simulink library "SimplusGT_2020a"  (R2021a)
settings: Solver=ode45  StartTime=0.0  StopTime=10.0  RelTol=1e-3
undefined symbols (not defined in the file): ang_r, Cf, DiscIntNeverNeededParam, initial, Lc, Lf, m, OtherInputs, P_dc, Sbase, t0, Tm_pu, Ts, V, Vbase, w_droop, w_i, w_pll, w_tau, w_v, Wbase, wc, wfil, x0, Ybase, Zbase
libraries: spsVoltageMeasurementLib x83, spsCurrentMeasurementLib x71, spsControlledCurrentSourceLib x33, spsThreePhaseSeriesRLCBranchLib x21, spsControlledVoltageSourceLib x19, spsSeriesRLCBranchLib x15, spsThreePhaseParallelRLCBranchLib x3, spsThreePhaseBreakerLib x2, $bdroot x1, SimplexPS_2015a x1
(part 3 of 6)

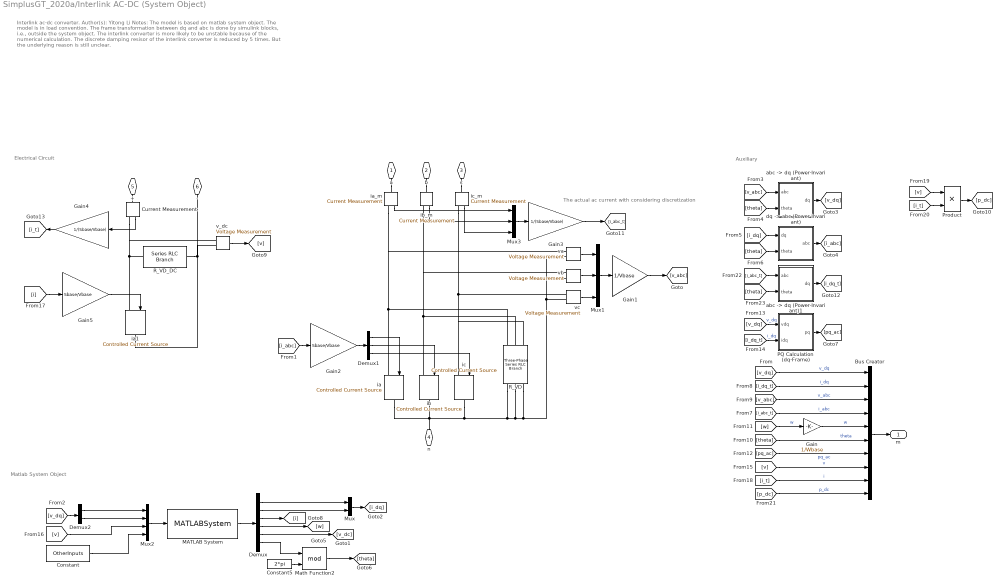
== system SimplusGT_2020a/Interlink AC-DC (System Object) ==
  note: Matlab System Object
  note: Auxiliary
  note: Electrical Circuit
  note: Interlink ac-dc converter.
      |
      | Author(s): Yitong Li
      |
      | Notes:
      |
      | The model is based on matlab system object.
      |
      | The model is in load convention.
      |
      | The frame transformation between dq and abc is done by simulink blocks, i.e., outside the system object.
      |
      | The interlink converter is more likely to be unstable because of the numerical calculation. The discrete damping resisor of the interlink converter is reduced by 5 times. But the underlying reason is still unclear.
  note: The actual ac current with considering discretization
  Bus Creator : BusCreator  Inputs=10
  Constant : Constant  Value=OtherInputs
  Constant5 : Constant  Value=2*pi
  Current Measurement : spsCurrentMeasurementLib/Current Measurement  PhasorSimulation=off  OutputType=Complex  PSBequivalent=0
  Demux : Demux  Outputs=6
  Demux1 : Demux  Outputs=3
  Demux2 : Demux  Outputs=2
  Gain : Gain  Gain=1/Wbase
  Gain1 : Gain  Gain=1/Vbase
  Gain2 : Gain  Gain=Sbase/Vbase
  Gain3 : Gain  Gain=1/(Sbase/Vbase)
  Gain4 : Gain  Gain=1/(Sbase/Vbase)
  Gain5 : Gain  Gain=Sbase/Vbase
  MATLAB System : MATLABSystem  System=SimplusGT.Class.InterlinkAcDc  Ts=Ts  Para=ApparatusPara  ApparatusType=ApparatusType  PowerFlow=PowerFlow  x0=x0  DiscreMethod=DiscreMethod  LinearizationTimes=LinearizationTimes  DirectFeedthrough=DirectFeedthrough  VirtualResistor=DiscreDampingFlag  EquiInitial=true  ElecPortIOs=[ 1, 2, 3 ]  SimulateUsing=Code generation
      mask Type: SimplusGT.Class.InterlinkAcDc
      mask Display:
      | disp('InterlinkAcDc');
      | port_label('input',1,'u');
      | port_label('output',1,'y');
  Math Function2 : Math  Operator=mod  SignedPower=on  SaturateOnIntegerOverflow=on
  Mux : Mux  Inputs=2
  Mux1 : Mux  Inputs=3
  Mux2 : Mux
  Mux3 : Mux  Inputs=3
  PQ Calculation (dq-Frame) : Subsystem  AncestorBlock=|
      | SimplusGT/PQ Calculation
      | (dq-Frame)
  Product : Product
  R_VD : spsThreePhaseSeriesRLCBranchLib/Three-Phase Series RLC Branch  LConnTagsString=A|B|C  RConnTagsString=A|B|C  BranchType=R  Resistance=DiscreDampingValue*Vbase^2/Sbase/5  Inductance=1e-3  Capacitance=1e-6  Measurements=None
  R_VD_DC : spsSeriesRLCBranchLib/Series RLC Branch  LConnTagsString=__new0  RConnTagsString=__new0  BranchType=R  Resistance=DiscreDampingValue*Vbase^2/Sbase/5  Inductance=1e-3  SetiL0=off  InitialCurrent=0  Capacitance=1e-6  Setx0=off  InitialVoltage=0  Measurements=None
  "abc -> dq (Power-Invariant)" : Subsystem  AncestorBlock=|
      | SimplusGT/abc -> dq
      | (Power-Invariant)
  "abc -> dq (Power-Invariant)1" : Subsystem  AncestorBlock=|
      | SimplusGT/abc -> dq
      | (Power-Invariant)
  "dq -> abc (Power-Invariant)" : Subsystem  AncestorBlock=|
      | SimplusGT/dq -> abc
      | (Power-Invariant)
  ia : spsControlledCurrentSourceLib/Controlled Current Source  Initialize=on  Source_Type=AC  Amplitude=0  Phase=0  Frequency=0  Measurements=None
  ia1 : spsControlledCurrentSourceLib/Controlled Current Source  Initialize=on  Source_Type=AC  Amplitude=0  Phase=0  Frequency=0  Measurements=None
  ia_m : spsCurrentMeasurementLib/Current Measurement  PhasorSimulation=off  OutputType=Complex  PSBequivalent=0
  ib : spsControlledCurrentSourceLib/Controlled Current Source  Initialize=on  Source_Type=AC  Amplitude=0  Phase=0  Frequency=0  Measurements=None
  ib_m : spsCurrentMeasurementLib/Current Measurement  PhasorSimulation=off  OutputType=Complex  PSBequivalent=0
  ic : spsControlledCurrentSourceLib/Controlled Current Source  Initialize=on  Source_Type=AC  Amplitude=0  Phase=0  Frequency=0  Measurements=None
  ic_m : spsCurrentMeasurementLib/Current Measurement  PhasorSimulation=off  OutputType=Complex  PSBequivalent=0
  v_dc : spsVoltageMeasurementLib/Voltage Measurement  PhasorSimulation=off  OutputType=Complex  PSBequivalent=0
  va : spsVoltageMeasurementLib/Voltage Measurement  PhasorSimulation=off  OutputType=Complex  PSBequivalent=0
  vb : spsVoltageMeasurementLib/Voltage Measurement  PhasorSimulation=off  OutputType=Complex  PSBequivalent=0
  vc : spsVoltageMeasurementLib/Voltage Measurement  PhasorSimulation=off  OutputType=Complex  PSBequivalent=0
  a : PMIOPort  Side=Left
  b : PMIOPort  Port=2  Side=Left
  c : PMIOPort  Port=3  Side=Left
  n : PMIOPort  Port=4  Side=Left
  + : PMIOPort  Port=5  Side=Left
  - : PMIOPort  Port=6  Side=Left
  m : Outport
  wires:
  Demux/2 -> Mux/2
  Demux/1 -> Mux/1
  Mux/1 -> [i_dq]
  Demux1/1 -> ia/1
  Demux1/2 -> ib/1
  va/1 -> Mux1/1
  vb/1 -> Mux1/2
  Mux1/1 -> Gain1/1
  [v_dq] -> Demux2/1
  Demux2/1 -> Mux2/1
  Demux2/2 -> Mux2/2
  [v_dq] -> Bus Creator/1  "v_dq"
  [i_dq_t] -> Bus Creator/2  "i_dq"
  [v_abc] -> Bus Creator/3  "v_abc"
  [i_abc_t] -> Bus Creator/4  "i_abc"
  [theta] -> Bus Creator/6  "theta"
  [v_abc] -> "abc -> dq (Power-Invariant)"/1(abc)
  [theta] -> "abc -> dq (Power-Invariant)"/2(theta)
  "abc -> dq (Power-Invariant)"/1(dq) -> [v_dq]
  [i_dq] -> "dq -> abc (Power-Invariant)"/1(dq)
  [theta] -> "dq -> abc (Power-Invariant)"/2(theta)
  "dq -> abc (Power-Invariant)"/1(abc) -> [i_abc]
  Mux2/1 -> MATLAB System/1
  MATLAB System/1 -> Demux/1
  vc/1 -> Mux1/3
  Demux1/3 -> ic/1
  Constant5/1 -> Math Function2/2
  Math Function2/1 -> [theta]
  Bus Creator/1 -> m/1
  Constant/1 -> Mux2/4
  [w] -> Gain/1  "w"
  Gain/1 -> Bus Creator/5  "w"
  [i_abc] -> Gain2/1
  [pq_ac] -> Bus Creator/7  "pq_ac"
  [v_dq] -> PQ Calculation (dq-Frame)/1(vdq)  "v_dq"
  [i_dq_t] -> PQ Calculation (dq-Frame)/2(idq)  "i_dq"
  PQ Calculation (dq-Frame)/1(pq) -> [pq_ac]
  Gain2/1 -> Demux1/1
  Gain1/1 -> [v_abc]
  [v] -> Bus Creator/8  "v"
  Demux/4 -> [w]
  Demux/5 -> [v_dc]
  Demux/6 -> Math Function2/1
  [v] -> Mux2/3
  Demux/3 -> [i]
  v_dc/1 -> [v]
  [i_t] -> Bus Creator/9  "i"
  [v] -> Product/1
  [i_t] -> Product/2
  Product/1 -> [p_dc]
  [p_dc] -> Bus Creator/10  "p_dc"
  ic_m/1 -> Mux3/3
  ib_m/1 -> Mux3/2
  Gain3/1 -> [i_abc_t]
  Mux3/1 -> Gain3/1
  ia_m/1 -> Mux3/1
  [theta] -> "abc -> dq (Power-Invariant)1"/2(theta)
  [i_abc_t] -> "abc -> dq (Power-Invariant)1"/1(abc)
  "abc -> dq (Power-Invariant)1"/1(dq) -> [i_dq_t]
  Gain4/1 -> [i_t]
  Current Measurement/1 -> Gain4/1
  [i] -> Gain5/1
  Gain5/1 -> ia1/1
  connections:
  vb/LConn2 -- va/LConn2 -- vc/LConn2 -- R_VD/RConn3 -- R_VD/RConn2 -- R_VD/RConn1 -- ic/RConn1 -- ia/RConn1 -- ib/RConn1 -- n/RConn1
  R_VD/LConn1 -- ia_m/RConn1 -- va/LConn1 -- ia/LConn1
  R_VD/LConn2 -- ib_m/RConn1 -- vb/LConn1 -- ib/LConn1
  R_VD/LConn3 -- ic/LConn1 -- ic_m/RConn1 -- vc/LConn1
  ia1/LConn1 -- Current Measurement/RConn1 -- v_dc/LConn1 -- R_VD_DC/LConn1
  ia1/RConn1 -- R_VD_DC/RConn1 -- -/RConn1 -- v_dc/LConn2
  c/RConn1 -- ic_m/LConn1
  b/RConn1 -- ib_m/LConn1
  a/RConn1 -- ia_m/LConn1
  Current Measurement/LConn1 -- +/RConn1

== system SimplusGT_2020a/L Filter (3ph) ==
  note: Model for a L filter.
      |
      | Author(s): Yitong Li
      |
      | Notes:
      |
      | vi is the converter side voltage, and vg is the grid side voltage.
  Bus Creator : BusCreator  Inputs=3
  "LL -> LN" : Subsystem
  "LL -> LN1" : Subsystem
  Mux : Mux  Inputs=3
  Mux1 : Mux  Inputs=3
  Mux2 : Mux  Inputs=3
  Three-Phase Series RLC Branch : spsThreePhaseSeriesRLCBranchLib/Three-Phase Series RLC Branch  LConnTagsString=A|B|C  RConnTagsString=A|B|C  BranchType=RL  Resistance=Rf  Inductance=Lf  Capacitance=1e-6  Measurements=None
  Vab : spsVoltageMeasurementLib/Voltage Measurement  PhasorSimulation=off  OutputType=Complex  PSBequivalent=0
  Vab1 : spsVoltageMeasurementLib/Voltage Measurement  PhasorSimulation=off  OutputType=Complex  PSBequivalent=0
  Vbc : spsVoltageMeasurementLib/Voltage Measurement  PhasorSimulation=off  OutputType=Complex  PSBequivalent=0
  Vbc1 : spsVoltageMeasurementLib/Voltage Measurement  PhasorSimulation=off  OutputType=Complex  PSBequivalent=0
  Vca : spsVoltageMeasurementLib/Voltage Measurement  PhasorSimulation=off  OutputType=Complex  PSBequivalent=0
  Vca1 : spsVoltageMeasurementLib/Voltage Measurement  PhasorSimulation=off  OutputType=Complex  PSBequivalent=0
  ila : spsCurrentMeasurementLib/Current Measurement  PhasorSimulation=off  OutputType=Complex  PSBequivalent=0
  ilb : spsCurrentMeasurementLib/Current Measurement  PhasorSimulation=off  OutputType=Complex  PSBequivalent=0
  ilc : spsCurrentMeasurementLib/Current Measurement  PhasorSimulation=off  OutputType=Complex  PSBequivalent=0
  via : PMIOPort  Side=Left
  vib : PMIOPort  Port=2  Side=Left
  vic : PMIOPort  Port=3  Side=Left
  vga : PMIOPort  Port=4  Side=Right
  vgb : PMIOPort  Port=5  Side=Right
  vgc : PMIOPort  Port=6  Side=Right
  m : Outport
  wires:
  Vab/1 -> Mux/1
  Vbc/1 -> Mux/2
  ilb/1 -> Mux2/2
  Vca/1 -> Mux/3
  Vca1/1 -> Mux1/3
  "LL -> LN1"/1(Out1) -> [vgabc]
  ilc/1 -> Mux2/3
  "LL -> LN"/1(Out1) -> [viabc]
  Mux1/1 -> "LL -> LN"/1(In1)
  Mux/1 -> "LL -> LN1"/1(In1)
  Vab1/1 -> Mux1/1
  ila/1 -> Mux2/1
  Mux2/1 -> [ilabc]
  Vbc1/1 -> Mux1/2
  [viabc] -> Bus Creator/1  "viabc"
  Bus Creator/1 -> m/1
  [vgabc] -> Bus Creator/2  "vgabc"
  [ilabc] -> Bus Creator/3  "ilabc"
  connections:
  Vca/LConn1 -- Vbc/LConn2 -- ilc/RConn1 -- vgc/RConn1
  Three-Phase Series RLC Branch/LConn1 -- via/RConn1 -- Vab1/LConn1 -- Vca1/LConn2
  Three-Phase Series RLC Branch/RConn2 -- ilb/LConn1
  Three-Phase Series RLC Branch/RConn3 -- ilc/LConn1
  Vab/LConn2 -- Vbc/LConn1 -- vgb/RConn1 -- ilb/RConn1
  Vbc1/LConn2 -- vic/RConn1 -- Three-Phase Series RLC Branch/LConn3 -- Vca1/LConn1
  Vab1/LConn2 -- vib/RConn1 -- Three-Phase Series RLC Branch/LConn2 -- Vbc1/LConn1
  Vca/LConn2 -- Vab/LConn1 -- ila/RConn1 -- vga/RConn1
  Three-Phase Series RLC Branch/RConn1 -- ila/LConn1

== system SimplusGT_2020a/LC Filter (3ph) ==
  note: Model for a LC filter.
      |
      | Author(s): Yitong Li
      |
      | Notes:
      |
      | vi is the converter side voltage, and vg is the grid side voltage.
  Bus Creator : BusCreator  Inputs=4
  "LL -> LN" : Subsystem
  Mux{1..4} (4 alike) : Mux  Inputs=3
  Three-Phase Series RLC Branch : spsThreePhaseSeriesRLCBranchLib/Three-Phase Series RLC Branch  LConnTagsString=A|B|C  RConnTagsString=A|B|C  BranchType=RL  Resistance=Rf  Inductance=Lf  Capacitance=1e-6  Measurements=None
  Three-Phase Series RLC Branch2 : spsThreePhaseSeriesRLCBranchLib/Three-Phase Series RLC Branch  LConnTagsString=A|B|C  RConnTagsString=A|B|C  BranchType=RC  Resistance=Rd  Inductance=Lc  Capacitance=Cf  Measurements=None
  Vab1 : spsVoltageMeasurementLib/Voltage Measurement  PhasorSimulation=off  OutputType=Complex  PSBequivalent=0
  Vbc1 : spsVoltageMeasurementLib/Voltage Measurement  PhasorSimulation=off  OutputType=Complex  PSBequivalent=0
  Vca1 : spsVoltageMeasurementLib/Voltage Measurement  PhasorSimulation=off  OutputType=Complex  PSBequivalent=0
  iga : spsCurrentMeasurementLib/Current Measurement  PhasorSimulation=off  OutputType=Complex  PSBequivalent=0
  igb : spsCurrentMeasurementLib/Current Measurement  PhasorSimulation=off  OutputType=Complex  PSBequivalent=0
  igc : spsCurrentMeasurementLib/Current Measurement  PhasorSimulation=off  OutputType=Complex  PSBequivalent=0
  ila : spsCurrentMeasurementLib/Current Measurement  PhasorSimulation=off  OutputType=Complex  PSBequivalent=0
  ilb : spsCurrentMeasurementLib/Current Measurement  PhasorSimulation=off  OutputType=Complex  PSBequivalent=0
  ilc : spsCurrentMeasurementLib/Current Measurement  PhasorSimulation=off  OutputType=Complex  PSBequivalent=0
  vca measure : spsVoltageMeasurementLib/Voltage Measurement  PhasorSimulation=off  OutputType=Complex  PSBequivalent=0
  vcb measure : spsVoltageMeasurementLib/Voltage Measurement  PhasorSimulation=off  OutputType=Complex  PSBequivalent=0
  vcc measure : spsVoltageMeasurementLib/Voltage Measurement  PhasorSimulation=off  OutputType=Complex  PSBequivalent=0
  via : PMIOPort  Side=Left
  vib : PMIOPort  Port=2  Side=Left
  vic : PMIOPort  Port=3  Side=Left
  vga : PMIOPort  Port=4  Side=Right
  vgb : PMIOPort  Port=5  Side=Right
  vgc : PMIOPort  Port=6  Side=Right
  N : PMIOPort  Port=7  Side=Left
  m : Outport
  wires:
  igb/1 -> Mux4/2
  iga/1 -> Mux4/1
  Vab1/1 -> Mux1/1
  vcb measure/1 -> Mux3/2
  [viabc] -> Bus Creator/1  "viabc"
  ilc/1 -> Mux2/3
  igc/1 -> Mux4/3
  ila/1 -> Mux2/1
  Mux1/1 -> "LL -> LN"/1(In1)
  Bus Creator/1 -> m/1
  vcc measure/1 -> Mux3/3
  ilb/1 -> Mux2/2
  vca measure/1 -> Mux3/1
  Mux3/1 -> [vcabc]
  "LL -> LN"/1(Out1) -> [viabc]
  Vca1/1 -> Mux1/3
  [vcabc] -> Bus Creator/2  "vcabc"
  Mux2/1 -> [ilabc]
  Mux4/1 -> [igabc]
  Vbc1/1 -> Mux1/2
  [ilabc] -> Bus Creator/3  "ilabc"
  [igabc] -> Bus Creator/4  "igabc"
  connections:
  Three-Phase Series RLC Branch2/LConn3 -- igc/LConn1 -- ilc/RConn1 -- vcc measure/LConn1
  Vbc1/LConn2 -- vic/RConn1 -- Three-Phase Series RLC Branch/LConn3 -- Vca1/LConn1
  Three-Phase Series RLC Branch/RConn3 -- ilc/LConn1
  vca measure/LConn1 -- ila/RConn1 -- iga/LConn1 -- Three-Phase Series RLC Branch2/LConn1
  vga/RConn1 -- iga/RConn1
  vgb/RConn1 -- igb/RConn1
  vcb measure/LConn1 -- igb/LConn1 -- ilb/RConn1 -- Three-Phase Series RLC Branch2/LConn2
  Vab1/LConn2 -- vib/RConn1 -- Three-Phase Series RLC Branch/LConn2 -- Vbc1/LConn1
  vgc/RConn1 -- igc/RConn1
  vcc measure/LConn2 -- vca measure/LConn2 -- vcb measure/LConn2 -- N/RConn1 -- Three-Phase Series RLC Branch2/RConn1 -- Three-Phase Series RLC Branch2/RConn2 -- Three-Phase Series RLC Branch2/RConn3
  Three-Phase Series RLC Branch/LConn1 -- via/RConn1 -- Vab1/LConn1 -- Vca1/LConn2
  Three-Phase Series RLC Branch/RConn1 -- ila/LConn1
  Three-Phase Series RLC Branch/RConn2 -- ilb/LConn1

== system SimplusGT_2020a/LCL Filter (3ph) ==
  note: Model for a LCL filter.
      |
      | Author(s): Yitong Li
      |
      | Notes:
      |
      | vi is the converter side voltage, and vg is the grid side voltage.
  Bus Creator : BusCreator  Inputs=5
  "LL -> LN" : Subsystem
  "LL -> LN1" : Subsystem
  Mux{,1..4} (5 alike) : Mux  Inputs=3
  Three-Phase Series RLC Branch : spsThreePhaseSeriesRLCBranchLib/Three-Phase Series RLC Branch  LConnTagsString=A|B|C  RConnTagsString=A|B|C  BranchType=RL  Resistance=Rf  Inductance=Lf  Capacitance=1e-6  Measurements=None
  Three-Phase Series RLC Branch1 : spsThreePhaseSeriesRLCBranchLib/Three-Phase Series RLC Branch  LConnTagsString=A|B|C  RConnTagsString=A|B|C  BranchType=RL  Resistance=Rc  Inductance=Lc  Capacitance=1e-6  Measurements=None
  Three-Phase Series RLC Branch2 : spsThreePhaseSeriesRLCBranchLib/Three-Phase Series RLC Branch  LConnTagsString=A|B|C  RConnTagsString=A|B|C  BranchType=RC  Resistance=Rd  Inductance=Lc  Capacitance=Cf  Measurements=None
  Vab : spsVoltageMeasurementLib/Voltage Measurement  PhasorSimulation=off  OutputType=Complex  PSBequivalent=0
  Vab1 : spsVoltageMeasurementLib/Voltage Measurement  PhasorSimulation=off  OutputType=Complex  PSBequivalent=0
  Vbc : spsVoltageMeasurementLib/Voltage Measurement  PhasorSimulation=off  OutputType=Complex  PSBequivalent=0
  Vbc1 : spsVoltageMeasurementLib/Voltage Measurement  PhasorSimulation=off  OutputType=Complex  PSBequivalent=0
  Vca : spsVoltageMeasurementLib/Voltage Measurement  PhasorSimulation=off  OutputType=Complex  PSBequivalent=0
  Vca1 : spsVoltageMeasurementLib/Voltage Measurement  PhasorSimulation=off  OutputType=Complex  PSBequivalent=0
  iga : spsCurrentMeasurementLib/Current Measurement  PhasorSimulation=off  OutputType=Complex  PSBequivalent=0
  igb : spsCurrentMeasurementLib/Current Measurement  PhasorSimulation=off  OutputType=Complex  PSBequivalent=0
  igc : spsCurrentMeasurementLib/Current Measurement  PhasorSimulation=off  OutputType=Complex  PSBequivalent=0
  ila : spsCurrentMeasurementLib/Current Measurement  PhasorSimulation=off  OutputType=Complex  PSBequivalent=0
  ilb : spsCurrentMeasurementLib/Current Measurement  PhasorSimulation=off  OutputType=Complex  PSBequivalent=0
  ilc : spsCurrentMeasurementLib/Current Measurement  PhasorSimulation=off  OutputType=Complex  PSBequivalent=0
  vca measure : spsVoltageMeasurementLib/Voltage Measurement  PhasorSimulation=off  OutputType=Complex  PSBequivalent=0
  vcb measure : spsVoltageMeasurementLib/Voltage Measurement  PhasorSimulation=off  OutputType=Complex  PSBequivalent=0
  vcc measure : spsVoltageMeasurementLib/Voltage Measurement  PhasorSimulation=off  OutputType=Complex  PSBequivalent=0
  via : PMIOPort  Side=Left
  vib : PMIOPort  Port=2  Side=Left
  vic : PMIOPort  Port=3  Side=Left
  vga : PMIOPort  Port=4  Side=Right
  vgb : PMIOPort  Port=5  Side=Right
  vgc : PMIOPort  Port=6  Side=Right
  N : PMIOPort  Port=7  Side=Left
  m : Outport
  wires:
  Mux4/1 -> [igabc]
  ilb/1 -> Mux2/2
  ila/1 -> Mux2/1
  igc/1 -> Mux4/3
  vcc measure/1 -> Mux3/3
  Vab/1 -> Mux/1
  Mux/1 -> "LL -> LN1"/1(In1)
  vca measure/1 -> Mux3/1
  vcb measure/1 -> Mux3/2
  igb/1 -> Mux4/2
  iga/1 -> Mux4/1
  Vca/1 -> Mux/3
  ilc/1 -> Mux2/3
  Vbc/1 -> Mux/2
  Mux2/1 -> [ilabc]
  Bus Creator/1 -> m/1
  "LL -> LN1"/1(Out1) -> [vgabc]
  Mux3/1 -> [vcabc]
  Vbc1/1 -> Mux1/2
  Vca1/1 -> Mux1/3
  Mux1/1 -> "LL -> LN"/1(In1)
  Vab1/1 -> Mux1/1
  "LL -> LN"/1(Out1) -> [viabc]
  [viabc] -> Bus Creator/1  "viabc"
  [vcabc] -> Bus Creator/2  "vcabc"
  [vgabc] -> Bus Creator/3  "vgabc"
  [ilabc] -> Bus Creator/4  "ilabc"
  [igabc] -> Bus Creator/5  "igabc"
  connections:
  vca measure/LConn2 -- Three-Phase Series RLC Branch2/RConn1 -- Three-Phase Series RLC Branch2/RConn2 -- N/RConn1 -- Three-Phase Series RLC Branch2/RConn3 -- vcc measure/LConn2 -- vcb measure/LConn2
  igc/RConn1 -- Vca/LConn1 -- Vbc/LConn2 -- vgc/RConn1
  Vbc1/LConn2 -- Three-Phase Series RLC Branch/LConn3 -- vic/RConn1 -- Vca1/LConn1
  Vab1/LConn2 -- vib/RConn1 -- Three-Phase Series RLC Branch/LConn2 -- Vbc1/LConn1
  Vca1/LConn2 -- Three-Phase Series RLC Branch/LConn1 -- via/RConn1 -- Vab1/LConn1
  ilc/RConn1 -- Three-Phase Series RLC Branch1/LConn3 -- vcc measure/LConn1 -- Three-Phase Series RLC Branch2/LConn3
  Three-Phase Series RLC Branch1/RConn2 -- igb/LConn1
  igb/RConn1 -- vgb/RConn1 -- Vbc/LConn1 -- Vab/LConn2
  vcb measure/LConn1 -- ilb/RConn1 -- Three-Phase Series RLC Branch1/LConn2 -- Three-Phase Series RLC Branch2/LConn2
  vca measure/LConn1 -- ila/RConn1 -- Three-Phase Series RLC Branch1/LConn1 -- Three-Phase Series RLC Branch2/LConn1
  Vca/LConn2 -- Vab/LConn1 -- vga/RConn1 -- iga/RConn1
  Three-Phase Series RLC Branch1/RConn1 -- iga/LConn1
  Three-Phase Series RLC Branch1/RConn3 -- igc/LConn1
  Three-Phase Series RLC Branch/RConn1 -- ila/LConn1
  Three-Phase Series RLC Branch/RConn2 -- ilb/LConn1
  Three-Phase Series RLC Branch/RConn3 -- ilc/LConn1

== system SimplusGT_2020a/LL -> LN ==
  note: Transformation from line-to-line voltage to line-to-neutral voltage.
      |
      | Author(s): Yitong Li
  In1 : Inport
  Fcn : Fcn  Expr=u[1]-u[3]
  Fcn1 : Fcn  Expr=u[2]-u[1]
  Fcn2 : Fcn  Expr=u[3]-u[2]
  Gain : Gain  Gain=1/3
  Mux9 : Mux  Inputs=3
  Out1 : Outport
  wires:
  Fcn/1 -> Mux9/1
  Fcn1/1 -> Mux9/2
  Fcn2/1 -> Mux9/3
  Mux9/1 -> Out1/1
  Gain/1 -> Fcn2/1, Fcn1/1, Fcn/1
  In1/1 -> Gain/1

== system SimplusGT_2020a/Load Impulse ==
  note: Model for an impulse load.
      |
      | Author(s): Yitong Li
  Single Pulse : $bdroot/Single Pulse  t0=t0  dt=dt  Am=1
  Three-Phase Breaker : spsThreePhaseBreakerLib/Three-Phase Breaker  InitialState=open  SwitchA=on  SwitchB=on  SwitchC=on  SwitchTimes="[1/60  5/60]"  External=on  BreakerResistance=R*1e-3  SnubberResistance=1e9  SnubberCapacitance=inf  Measurements=None
  load : spsThreePhaseParallelRLCBranchLib/Three-Phase Parallel RLC Branch  LConnTagsString=A|B|C  RConnTagsString=A|B|C  BranchType=R  Resistance=R  Inductance=1  Capacitance=1  Measurements=None
      settings: SourceProductBaseCode=PS
  a : PMIOPort  Side=Left
  b : PMIOPort  Port=2  Side=Left
  c : PMIOPort  Port=3  Side=Left
  n : PMIOPort  Port=4  Side=Right
  wires:
  Single Pulse/1 -> Three-Phase Breaker/1
  connections:
  load/RConn2 -- load/RConn3 -- load/RConn1 -- n/RConn1
  Three-Phase Breaker/RConn1 -- load/LConn3
  Three-Phase Breaker/RConn2 -- load/LConn2
  Three-Phase Breaker/RConn3 -- load/LConn1
  c/RConn1 -- Three-Phase Breaker/LConn1
  b/RConn1 -- Three-Phase Breaker/LConn2
  a/RConn1 -- Three-Phase Breaker/LConn3

== system SimplusGT_2020a/Load Step ==
  note: Model for a step load.
      |
      | Author(s): Yitong Li
  Constant : Constant  Value=Reverse
  Step : Step  Time=t0  SampleTime=0
  Step1 : Step  Time=t0  Before=1  After=0  SampleTime=0
  Switch : Switch  Criteria=u2 > Threshold  Threshold=0.5
  Three-Phase Breaker : spsThreePhaseBreakerLib/Three-Phase Breaker  InitialState=open  SwitchA=on  SwitchB=on  SwitchC=on  SwitchTimes="[1/60  5/60]"  External=on  BreakerResistance=R*1e-3  SnubberResistance=1e9  SnubberCapacitance=inf  Measurements=None
  load : spsThreePhaseParallelRLCBranchLib/Three-Phase Parallel RLC Branch  LConnTagsString=A|B|C  RConnTagsString=A|B|C  BranchType=R  Resistance=R  Inductance=1  Capacitance=1  Measurements=None
      settings: SourceProductBaseCode=PS
  a : PMIOPort  Side=Left
  b : PMIOPort  Port=2  Side=Left
  c : PMIOPort  Port=3  Side=Left
  n : PMIOPort  Port=4  Side=Right
  wires:
  Switch/1 -> Three-Phase Breaker/1
  Constant/1 -> Switch/2
  Step1/1 -> Switch/1
  Step/1 -> Switch/3
  connections:
  a/RConn1 -- Three-Phase Breaker/LConn3
  b/RConn1 -- Three-Phase Breaker/LConn2
  Three-Phase Breaker/RConn3 -- load/LConn1
  Three-Phase Breaker/RConn2 -- load/LConn2
  load/RConn2 -- n/RConn1 -- load/RConn3 -- load/RConn1
  Three-Phase Breaker/RConn1 -- load/LConn3
  c/RConn1 -- Three-Phase Breaker/LConn1

== system SimplusGT_2020a/P-w droop ==
  note: p-w droop controller
      |
      | Author(s): Yitong Li
      |
      | Notes:
      |
      | The power reference should be in source convention.
  pq : Inport
  Constant : Constant  Value=w0
  Constant2 : Constant  Value=theta0
  Constant4 : Constant  Value=2*pi
  Constant6 : Constant  Value=p0
  Demux : Demux  Outputs=2
  Discrete-Time Integrator : DiscreteIntegrator  SampleTime=Ts  ICPrevOutput=DiscIntNeverNeededParam  ICPrevScaledInput=DiscIntNeverNeededParam
  Filter p : DiscreteTransferFcn  Numerator=w_tau*Ts  Denominator=[1 ((w_tau*Ts)-1)]  SampleTime=Ts
  Gain : Gain  Gain=1/Sbase
  Gain2 : Gain  Gain=m
  Gain3 : Gain  Gain=Wbase
  Math Function1 : Math  Operator=mod  SignedPower=on  SaturateOnIntegerOverflow=on
  Sum : Sum
  Sum1 : Sum
  Sum2 : Sum  Inputs=+-
  w : Outport
  theta : Outport  Port=2
  wires:
  Gain3/1 -> Discrete-Time Integrator/1, w/1, [w]
  Sum/1 -> Gain3/1
  Sum2/1 -> Gain2/1
  Constant6/1 -> Sum2/1
  pq/1 -> Demux/1
  Constant4/1 -> Math Function1/2
  Constant/1 -> Sum/2
  Filter p/1 -> Sum2/2
  Discrete-Time Integrator/1 -> Sum1/1
  Gain2/1 -> Sum/1
  Math Function1/1 -> theta/1, [theta]
  Constant2/1 -> [theta0], Sum1/2
  Sum1/1 -> Math Function1/1
  Demux/1 -> Gain/1  "p"
  Gain/1 -> Filter p/1

== system SimplusGT_2020a/PLL (vDQ -> vq) ==
  note: Gpll
  note: Measurement
  note: Phase lock loop (PLL)
      |
      | Author(s): Yitong Li
      |
      | Notes:
      |
      | vq is fed into the PI controller of the PLL.
      |
      | This PLL assumes the input voltage is in DQ frame, which is the common electrical frame. It is not a practical PLL which uses vabc as the input. But this PLL is useful in research.
  vDQ : Inport
  wDQ : Inport  Port=2
  Constant1 : Constant
  Constant2 : Constant  Value=theta0
  Constant3 : Constant
  Constant4 : Constant  Value=2*pi
  Constant6 : Constant  Value=0
  Demux1 : Demux  Outputs=2
  Discrete PI1 : Subsystem  AncestorBlock=SimplusGT/Discrete PI  mask{Kp=w_pll, Ki=w_pll*w_pll/4, xmax=inf, xmin=-inf, Ts=Ts}
      mask prompts: Kp "Proportional Gain"; Ki "Integral Gain"; xmax "Upper Limit"; xmin "Lower Limit"; Ts "Sampling Time"
  Discrete-Time Integrator : DiscreteIntegrator  SampleTime=Ts  ICPrevOutput=DiscIntNeverNeededParam  ICPrevScaledInput=DiscIntNeverNeededParam
  Filter p : DiscreteTransferFcn  Numerator=w_tau*Ts  Denominator=[1 ((w_tau*Ts)-1)]  SampleTime=Ts
  Gain1 : Gain  Gain=Wbase
  Gain2 : Gain  Gain=1/Vbase
  Gain4 : Gain  Gain=1/Wbase
  Gain5 : Gain  Gain=1/pi
  Math Function1 : Math  Operator=mod  SignedPower=on  SaturateOnIntegerOverflow=on
  Mux : Mux  Inputs=2
  Scope : Scope  NumInputPorts=4
  Sum : Sum
  Sum1 : Sum
  Sum2 : Sum  Inputs=+-
  "x1y1 -> x2y2" : Subsystem  AncestorBlock=SimplusGT/x1y1 -> x2y2
  wdq : Outport
  theta : Outport  Port=2
  vdq : Outport  Port=3
  wires:
  [theta0] -> Mux/1  "theta0"
  Constant2/1 -> [theta0], Sum1/2
  Math Function1/1 -> "x1y1 -> x2y2"/2(theta), theta/1, [theta]
  Sum1/1 -> Math Function1/1
  Demux1/2 -> [vq], Gain2/1
  vDQ/1 -> "x1y1 -> x2y2"/1(x1y1)
  Discrete-Time Integrator/1 -> Sum1/1
  Gain2/1 -> Filter p/1
  [vd] -> Scope/1  "vd"
  Mux/1 -> Gain5/1
  Discrete PI1/1(Out) -> Sum/1
  "x1y1 -> x2y2"/1(x2y2) -> vdq/1, Demux1/1
  [w] -> Gain4/1  "w"
  Constant4/1 -> Math Function1/2
  [theta] -> Mux/2  "theta"
  Demux1/1 -> [vd]
  Gain5/1 -> Scope/4
  Constant1/1 -> Discrete PI1/1(enable)
  Gain4/1 -> Scope/3
  Gain1/1 -> Sum/2
  Constant3/1 -> Gain1/1
  [vq] -> Scope/2  "vq"
  Filter p/1 -> Discrete PI1/2(reference)
  Constant6/1 -> Discrete PI1/4(actual), Discrete PI1/3(initial)
  Sum/1 -> Sum2/1
  Sum2/1 -> [w], wdq/1, Discrete-Time Integrator/1
  wDQ/1 -> Sum2/2

== system SimplusGT_2020a/PLL (vabc -> theta) ==
  note: Measurement
  note: Gpll
  note: Phase lock loop (PLL)
      |
      | Author(s): Yitong Li
      |
      | Notes:
      |
      | theta of voltage is fed into the PI controller of the PLL.
  vabc : Inport
  Constant1 : Constant
  Constant2 : Constant  Value=2*pi
  Constant3 : Constant  Value=0
  Constant4 : Constant
  Constant5 : Constant  Value=theta0
  Demux : Demux  Outputs=2
  Discrete PI : Subsystem  AncestorBlock=SimplusGT/Discrete PI  mask{Kp=w_pll, Ki=w_pll*w_pll/4, xmax=inf, xmin=-inf, Ts=Ts}
      mask prompts: Kp "Proportional Gain"; Ki "Integral Gain"; xmax "Upper Limit"; xmin "Lower Limit"; Ts "Sampling Time"
  Discrete-Time Integrator : DiscreteIntegrator  SampleTime=Ts  ICPrevOutput=DiscIntNeverNeededParam  ICPrevScaledInput=DiscIntNeverNeededParam
  Filter p : DiscreteTransferFcn  Numerator=w_tau*Ts  Denominator=[1 ((w_tau*Ts)-1)]  SampleTime=Ts
  Gain1 : Gain  Gain=Wbase
  Gain4 : Gain  Gain=1/Wbase
  Gain5 : Gain  Gain=1/pi
  Math Function1 : Math  Operator=mod  SignedPower=on  SaturateOnIntegerOverflow=on
  Mux : Mux  Inputs=2
  Scope : Scope  NumInputPorts=4
  Selector : Selector  InputPortWidth=2  IndexOptions=Index vector (dialog)  Indices=[2 1]  OutputSizes=1
  Sum : Sum
  Sum1 : Sum
  Trigonometric Function : Trigonometry  Operator=atan2
  "abc -> dq (Power-Invariant)" : Subsystem  AncestorBlock=|
      | SimplusGT/abc -> dq
      | (Power-Invariant)
  w : Outport
  theta : Outport  Port=2
  vdq : Outport  Port=3
  wires:
  Constant2/1 -> Math Function1/2
  Constant1/1 -> Discrete PI/1(enable)
  Constant3/1 -> Discrete PI/3(initial), Discrete PI/4(actual)
  Trigonometric Function/1 -> Filter p/1
  Demux/1 -> [vq], Trigonometric Function/1
  Demux/2 -> [vd], Trigonometric Function/2
  Selector/1 -> Demux/1
  Math Function1/1 -> "abc -> dq (Power-Invariant)"/2(theta), [theta], theta/1
  "abc -> dq (Power-Invariant)"/1(dq) -> vdq/1, Selector/1
  vabc/1 -> "abc -> dq (Power-Invariant)"/1(abc)
  Discrete PI/1(Out) -> Sum/1
  Constant4/1 -> Gain1/1
  Sum/1 -> [w], w/1, Discrete-Time Integrator/1
  Filter p/1 -> Discrete PI/2(reference)
  [vq] -> Scope/2  "vq"
  Mux/1 -> Gain5/1
  [vd] -> Scope/1  "vd"
  [theta] -> Mux/2  "theta"
  Gain5/1 -> Scope/4
  Gain4/1 -> Scope/3
  [w] -> Gain4/1  "w"
  [theta0] -> Mux/1  "theta0"
  Gain1/1 -> Sum/2
  Discrete-Time Integrator/1 -> Sum1/1
  Sum1/1 -> Math Function1/1
  Constant5/1 -> [theta0], Sum1/2

== system SimplusGT_2020a/PLL (vabc -> vd+jvq) ==
  note: Measurement
  note: Frame trabsformation
  note: -j
  note: Gpll
  note: Gpll
  note: Phase lock loop (PLL)
      |
      | Author(s): Yitong Li
      |
      | Notes:
      |
      | This is a symmetric PLL controls both d- and q-axis voltage.
      |
      | It is built based on Dongsheng Yang's paper: "Symmetrical PLL for SISO Impedance Modeling and Enhanced Stability in Weak Grids", IEEE Transactions on Power Electronics, 2020.
  vabc : Inport
  Constant{,2..3,7} (4 alike) : Constant
  Constant{1,5..6,8} (4 alike) : Constant  Value=0
  Constant10 : Constant  Value=theta_d0
  Constant4 : Constant  Value=2*pi
  Constant9 : Constant  Value=theta_q0
  Demux1 : Demux  Outputs=2
  Discrete PI_d : Subsystem  AncestorBlock=SimplusGT/Discrete PI  mask{Kp=w_pll, Ki=w_pll*w_pll/4, xmax=inf, xmin=-inf, Ts=Ts}
      mask prompts: Kp "Proportional Gain"; Ki "Integral Gain"; xmax "Upper Limit"; xmin "Lower Limit"; Ts "Sampling Time"
  Discrete PI_q : Subsystem  AncestorBlock=SimplusGT/Discrete PI  mask{Kp=w_pll, Ki=w_pll*w_pll/4, xmax=inf, xmin=-inf, Ts=Ts}
      mask prompts: Kp "Proportional Gain"; Ki "Integral Gain"; xmax "Upper Limit"; xmin "Lower Limit"; Ts "Sampling Time"
  Discrete-Time Integrator : DiscreteIntegrator  SampleTime=Ts  ICPrevOutput=DiscIntNeverNeededParam  ICPrevScaledInput=DiscIntNeverNeededParam
  Discrete-Time Integrator1 : DiscreteIntegrator  SampleTime=Ts  ICPrevOutput=DiscIntNeverNeededParam  ICPrevScaledInput=DiscIntNeverNeededParam
  Exp : Math  SignedPower=on  SaturateOnIntegerOverflow=on
  Filter p : DiscreteTransferFcn  Numerator=w_tau*Ts  Denominator=[1 ((w_tau*Ts)-1)]  SampleTime=Ts
  Filter p1 : DiscreteTransferFcn  Numerator=w_tau*Ts  Denominator=[1 ((w_tau*Ts)-1)]  SampleTime=Ts
  Gain : Gain  Gain=Wbase
  Gain1 : Gain  Gain=Wbase
  Gain2 : Gain  Gain=1/Wbase
  Gain3 : Gain  Gain=-1
  Gain4 : Gain  Gain=1/pi
  Gain5 : Gain  Gain=1/Vbase
  Math Function1 : Math  Operator=mod  SignedPower=on  SaturateOnIntegerOverflow=on
  Mux : Mux  Inputs=2
  Mux1 : Mux  Inputs=2
  Mux2 : Mux  Inputs=2
  Product : Product
  Scope : Scope  NumInputPorts=3
  Sum : Sum  Inputs=|+-
  Sum{1..2,4..5} (4 alike) : Sum
  Sum3 : Sum  Inputs=|+-
  "abc -> dq (Power-Invariant)" : Subsystem  AncestorBlock=|
      | SimplusGT/abc -> dq
      | (Power-Invariant)
  wd : Outport
  theta_d : Outport  Port=2
  wq : Outport  Port=3
  theta_q : Outport  Port=4
  wires:
  Constant4/1 -> Math Function1/2
  Constant6/1 -> Discrete PI_q/3(initial), Discrete PI_q/4(actual)
  Demux1/2 -> [vq]
  Constant3/1 -> Discrete PI_q/1(enable)
  Math Function1/1 -> theta_d/1, [thetad]
  "abc -> dq (Power-Invariant)"/1(dq) -> Gain5/1
  Gain5/1 -> Demux1/1
  Demux1/1 -> [vd]
  Constant/1 -> Sum/2
  Sum/1 -> Discrete PI_d/2(reference)
  Constant7/1 -> Discrete PI_d/1(enable)
  Constant1/1 -> Discrete PI_d/4(actual), Discrete PI_d/3(initial)
  [thetad] -> "abc -> dq (Power-Invariant)"/2(theta)
  vabc/1 -> Product/1
  Product/1 -> "abc -> dq (Power-Invariant)"/1(abc)
  Exp/1 -> Product/2
  Gain3/1 -> theta_q/1, [thetaq]
  [vq] -> Filter p/1
  [vd] -> Filter p1/1
  Filter p1/1 -> Sum/1
  [thetaq] -> Exp/1
  Sum1/1 -> [wd], wd/1, Discrete-Time Integrator/1
  Discrete PI_q/1(Out) -> Sum1/1
  Sum2/1 -> Discrete-Time Integrator1/1, wq/1, [wq]
  Discrete PI_d/1(Out) -> Sum2/1
  Constant2/1 -> Gain/1
  Constant5/1 -> Gain1/1
  Filter p/1 -> Sum3/1
  Constant8/1 -> Sum3/2
  Sum3/1 -> Discrete PI_q/2(reference)
  Discrete-Time Integrator1/1 -> Sum4/1
  Sum4/1 -> Gain3/1
  Constant9/1 -> Sum4/2
  Gain/1 -> Sum1/2
  Gain1/1 -> Sum2/2
  Discrete-Time Integrator/1 -> Sum5/1
  Sum5/1 -> Math Function1/1
  Constant10/1 -> Sum5/2
  [vd] -> Mux/1
  [vq] -> Mux/2
  [wd] -> Mux1/1
  [wq] -> Mux1/2
  [thetad] -> Mux2/1
  [thetaq] -> Mux2/2
  Mux/1 -> Scope/1  "vdq"
  Mux1/1 -> Gain2/1  "wdq"
  Mux2/1 -> Gain4/1  "thetadq"
  Gain2/1 -> Scope/2
  Gain4/1 -> Scope/3

== system SimplusGT_2020a/PLL (vabc -> vq) ==
  note: Measurement
  note: Gpll
  note: Phase lock loop (PLL)
      |
      | Author(s): Yitong Li
      |
      | Notes:
      |
      | vq is fed into the PI controller of the PLL.
  vabc : Inport
  Constant1 : Constant
  Constant2 : Constant  Value=theta0
  Constant3 : Constant
  Constant4 : Constant  Value=2*pi
  Constant6 : Constant  Value=0
  Demux1 : Demux  Outputs=2
  Discrete PI : Subsystem  AncestorBlock=SimplusGT/Discrete PI  mask{Kp=w_pll, Ki=w_pll*w_pll/4, xmax=inf, xmin=-inf, Ts=Ts}
      mask prompts: Kp "Proportional Gain"; Ki "Integral Gain"; xmax "Upper Limit"; xmin "Lower Limit"; Ts "Sampling Time"
  Discrete-Time Integrator : DiscreteIntegrator  SampleTime=Ts  ICPrevOutput=DiscIntNeverNeededParam  ICPrevScaledInput=DiscIntNeverNeededParam
  Filter p : DiscreteTransferFcn  Numerator=w_tau*Ts  Denominator=[1 ((w_tau*Ts)-1)]  SampleTime=Ts
  Gain1 : Gain  Gain=Wbase
  Gain2 : Gain  Gain=1/Vbase
  Gain4 : Gain  Gain=1/Wbase
  Gain5 : Gain  Gain=1/pi
  Math Function1 : Math  Operator=mod  SignedPower=on  SaturateOnIntegerOverflow=on
  Mux : Mux  Inputs=2
  Scope : Scope  NumInputPorts=4
  Sum : Sum
  Sum1 : Sum
  "abc -> dq (Power-Invariant)" : Subsystem  AncestorBlock=|
      | SimplusGT/abc -> dq
      | (Power-Invariant)
  w : Outport
  theta : Outport  Port=2
  vdq : Outport  Port=3
  wires:
  vabc/1 -> "abc -> dq (Power-Invariant)"/1(abc)
  "abc -> dq (Power-Invariant)"/1(dq) -> vdq/1, Demux1/1
  Constant4/1 -> Math Function1/2
  Gain2/1 -> Filter p/1
  Demux1/2 -> [vq], Gain2/1
  Constant6/1 -> Discrete PI/4(actual), Discrete PI/3(initial)
  Constant1/1 -> Discrete PI/1(enable)
  Discrete PI/1(Out) -> Sum/1
  Sum/1 -> [w], w/1, Discrete-Time Integrator/1
  Gain1/1 -> Sum/2
  Discrete-Time Integrator/1 -> Sum1/1
  Sum1/1 -> Math Function1/1
  Constant2/1 -> [theta0], Sum1/2
  Filter p/1 -> Discrete PI/2(reference)
  [vq] -> Scope/2  "vq"
  Mux/1 -> Gain5/1
  Gain4/1 -> Scope/3
  [w] -> Gain4/1  "w"
  [theta0] -> Mux/1  "theta0"
  [vd] -> Scope/1  "vd"
  Gain5/1 -> Scope/4
  [theta] -> Mux/2  "theta"
  Demux1/1 -> [vd]
  Constant3/1 -> Gain1/1
  Math Function1/1 -> "abc -> dq (Power-Invariant)"/2(theta), [theta], theta/1

== system SimplusGT_2020a/PQ Calculation (dq-Frame) ==
  note: Power calculation.
      |
      | Author(s): Yitong Li
      |
      | Notes:
      |
      | The calculation is done in dq frame.
  vdq : Inport
  idq : Inport  Port=2
  Mux : Mux  Inputs=2
  Mux1 : Mux  Inputs=2
  P = vd*id+vq*iq : Fcn  Expr=u[1]*u[3]+u[2]*u[4]
  Q = -vd*iq+vq*id : Fcn  Expr=-u[1]*u[4]+u[2]*u[3]
  pq : Outport
  wires:
  Q = -vd*iq+vq*id/1 -> Mux/2
  Mux1/1 -> Q = -vd*iq+vq*id/1, P = vd*id+vq*iq/1
  idq/1 -> Mux1/2
  vdq/1 -> Mux1/1
  P = vd*id+vq*iq/1 -> Mux/1
  Mux/1 -> pq/1

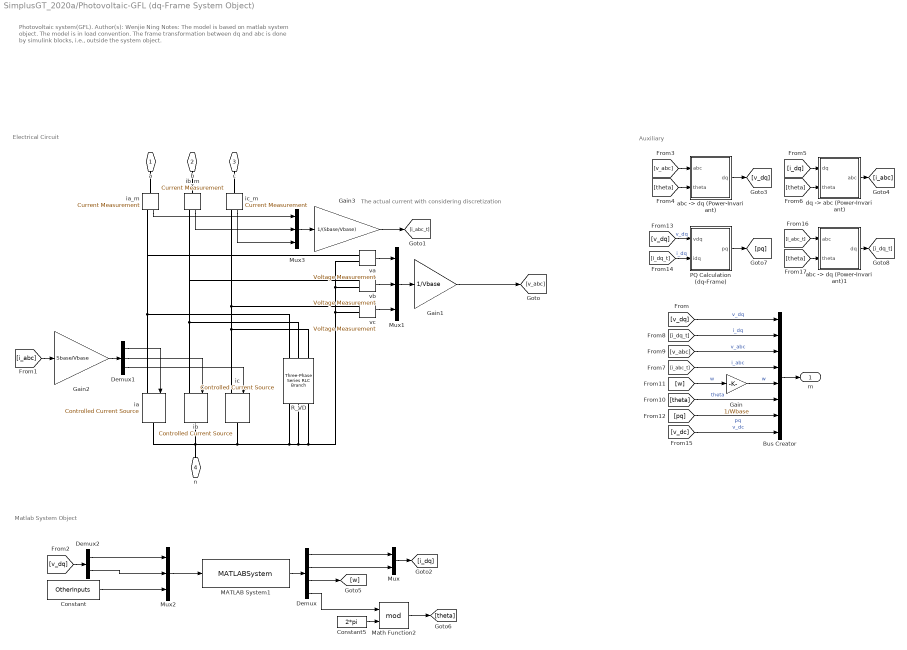
== system SimplusGT_2020a/Photovoltaic-GFL (dq-Frame System Object) ==
  note: Matlab System Object
  note: Auxiliary
  note: Electrical Circuit
  note: Photovoltaic system(GFL).
      |
      | Author(s): Wenjie Ning
      |
      | Notes:
      |
      | The model is based on matlab system object.
      |
      | The model is in load convention.
      |
      | The frame transformation between dq and abc is done by simulink blocks, i.e., outside the system object.
  note: The actual current with considering discretization
  Bus Creator : BusCreator  Inputs=8
  Constant : Constant  Value=OtherInputs
  Constant5 : Constant  Value=2*pi
  Demux : Demux
  Demux1 : Demux  Outputs=3
  Demux2 : Demux  Outputs=2
  Gain : Gain  Gain=1/Wbase
  Gain1 : Gain  Gain=1/Vbase
  Gain2 : Gain  Gain=Sbase/Vbase
  Gain3 : Gain  Gain=1/(Sbase/Vbase)
  MATLAB System1 : MATLABSystem  System=SimplusGT.Class.PhotovoltaicGFL  Ts=Ts  Para=ApparatusPara  ApparatusType=ApparatusType  PowerFlow=PowerFlow  x0=x0  DiscreMethod=DiscreMethod  LinearizationTimes=LinearizationTimes  DirectFeedthrough=DirectFeedthrough  VirtualResistor=DiscreDampingFlag  EquiInitial=true  ElecPortIOs=[ 1, 2 ]  SimulateUsing=Code generation
      mask Type: SimplusGT.Class.PhotovoltaicGFL
      mask Display:
      | disp('PhotovoltaicGFL');
      | port_label('input',1,'u');
      | port_label('output',1,'y');
  Math Function2 : Math  Operator=mod  SignedPower=on  SaturateOnIntegerOverflow=on
  Mux : Mux  Inputs=2
  Mux1 : Mux  Inputs=3
  Mux2 : Mux  Inputs=3
  Mux3 : Mux  Inputs=3
  PQ Calculation (dq-Frame) : Subsystem  AncestorBlock=|
      | SimplusGT/PQ Calculation
      | (dq-Frame)
  R_VD : spsThreePhaseSeriesRLCBranchLib/Three-Phase Series RLC Branch  LConnTagsString=A|B|C  RConnTagsString=A|B|C  BranchType=R  Resistance=DiscreDampingValue*Vbase^2/Sbase  Inductance=1e-3  Capacitance=1e-6  Measurements=None
  "abc -> dq (Power-Invariant)" : Subsystem  AncestorBlock=|
      | SimplusGT/abc -> dq
      | (Power-Invariant)
  "abc -> dq (Power-Invariant)1" : Subsystem  AncestorBlock=|
      | SimplusGT/abc -> dq
      | (Power-Invariant)
  "dq -> abc (Power-Invariant)" : Subsystem  AncestorBlock=|
      | SimplusGT/dq -> abc
      | (Power-Invariant)
  ia : spsControlledCurrentSourceLib/Controlled Current Source  Initialize=on  Source_Type=AC  Amplitude=0  Phase=0  Frequency=0  Measurements=None
  ia_m : spsCurrentMeasurementLib/Current Measurement  PhasorSimulation=off  OutputType=Complex  PSBequivalent=0
  ib : spsControlledCurrentSourceLib/Controlled Current Source  Initialize=on  Source_Type=AC  Amplitude=0  Phase=0  Frequency=0  Measurements=None
  ib_m : spsCurrentMeasurementLib/Current Measurement  PhasorSimulation=off  OutputType=Complex  PSBequivalent=0
  ic : spsControlledCurrentSourceLib/Controlled Current Source  Initialize=on  Source_Type=AC  Amplitude=0  Phase=0  Frequency=0  Measurements=None
  ic_m : spsCurrentMeasurementLib/Current Measurement  PhasorSimulation=off  OutputType=Complex  PSBequivalent=0
  va : spsVoltageMeasurementLib/Voltage Measurement  PhasorSimulation=off  OutputType=Complex  PSBequivalent=0
  vb : spsVoltageMeasurementLib/Voltage Measurement  PhasorSimulation=off  OutputType=Complex  PSBequivalent=0
  vc : spsVoltageMeasurementLib/Voltage Measurement  PhasorSimulation=off  OutputType=Complex  PSBequivalent=0
  a : PMIOPort  Side=Left
  b : PMIOPort  Port=2  Side=Left
  c : PMIOPort  Port=3  Side=Left
  n : PMIOPort  Port=4  Side=Left
  m : Outport
  wires:
  Demux/2 -> Mux/2
  Demux/1 -> Mux/1
  Mux/1 -> [i_dq]
  Demux/3 -> [w]
  Demux1/1 -> ia/1
  Demux1/2 -> ib/1
  va/1 -> Mux1/1
  vb/1 -> Mux1/2
  Mux1/1 -> Gain1/1
  [v_dq] -> Demux2/1
  Demux2/1 -> Mux2/1
  Demux2/2 -> Mux2/2
  [v_dq] -> Bus Creator/1  "v_dq"
  [i_dq_t] -> Bus Creator/2  "i_dq"
  [v_abc] -> Bus Creator/3  "v_abc"
  [i_abc_t] -> Bus Creator/4  "i_abc"
  [theta] -> Bus Creator/6  "theta"
  [v_abc] -> "abc -> dq (Power-Invariant)"/1(abc)
  [theta] -> "abc -> dq (Power-Invariant)"/2(theta)
  "abc -> dq (Power-Invariant)"/1(dq) -> [v_dq]
  [i_dq] -> "dq -> abc (Power-Invariant)"/1(dq)
  [theta] -> "dq -> abc (Power-Invariant)"/2(theta)
  "dq -> abc (Power-Invariant)"/1(abc) -> [i_abc]
  Mux2/1 -> MATLAB System1/1
  MATLAB System1/1 -> Demux/1
  vc/1 -> Mux1/3
  Demux1/3 -> ic/1
  Constant5/1 -> Math Function2/2
  Math Function2/1 -> [theta]
  Bus Creator/1 -> m/1
  [w] -> Gain/1  "w"
  Gain/1 -> Bus Creator/5  "w"
  [i_abc] -> Gain2/1
  [pq] -> Bus Creator/7  "pq"
  [v_dq] -> PQ Calculation (dq-Frame)/1(vdq)  "v_dq"
  [i_dq_t] -> PQ Calculation (dq-Frame)/2(idq)  "i_dq"
  PQ Calculation (dq-Frame)/1(pq) -> [pq]
  Gain2/1 -> Demux1/1
  Gain1/1 -> [v_abc]
  [v_dc] -> Bus Creator/8  "v_dc"
  Demux/4 -> Math Function2/1
  Constant/1 -> Mux2/3
  ic_m/1 -> Mux3/3
  ia_m/1 -> Mux3/1
  ib_m/1 -> Mux3/2
  Gain3/1 -> [i_abc_t]
  Mux3/1 -> Gain3/1
  [i_abc_t] -> "abc -> dq (Power-Invariant)1"/1(abc)
  [theta] -> "abc -> dq (Power-Invariant)1"/2(theta)
  "abc -> dq (Power-Invariant)1"/1(dq) -> [i_dq_t]
  connections:
  vb/LConn2 -- va/LConn2 -- vc/LConn2 -- R_VD/RConn3 -- R_VD/RConn2 -- R_VD/RConn1 -- ic/RConn1 -- ia/RConn1 -- ib/RConn1 -- n/RConn1
  R_VD/LConn1 -- va/LConn1 -- ia_m/RConn1 -- ia/LConn1
  R_VD/LConn2 -- ib_m/RConn1 -- vb/LConn1 -- ib/LConn1
  R_VD/LConn3 -- ic/LConn1 -- ic_m/RConn1 -- vc/LConn1
  ia_m/LConn1 -- a/RConn1
  ib_m/LConn1 -- b/RConn1
  ic_m/LConn1 -- c/RConn1

== system SimplusGT_2020a/Photovoltaic-GFM (dq-Frame System Object) ==
  note: The actual current with considering discretization
  note: Photovoltaic system(GFM).
      |
      | Author(s): Wenjie Ning
      |
      | Notes:
      |
      | The model is based on matlab system object.
      |
      | The model is in load convention.
      |
      | The frame transformation between dq and abc is done by simulink blocks, i.e., outside the system object.
  note: Electrical Circuit
  note: Auxiliary
  note: Matlab System Object
  Bus Creator : BusCreator  Inputs=8
  Constant : Constant  Value=OtherInputs
  Constant5 : Constant  Value=2*pi
  Demux : Demux
  Demux1 : Demux  Outputs=3
  Demux2 : Demux  Outputs=2
  Gain : Gain  Gain=1/Wbase
  Gain1 : Gain  Gain=1/Vbase
  Gain2 : Gain  Gain=Sbase/Vbase
  Gain3 : Gain  Gain=1/(Sbase/Vbase)
  MATLAB System : MATLABSystem  System=SimplusGT.Class.PhotovoltaicGFM  Ts=Ts  Para=ApparatusPara  ApparatusType=ApparatusType  PowerFlow=PowerFlow  x0=x0  DiscreMethod=DiscreMethod  LinearizationTimes=LinearizationTimes  DirectFeedthrough=DirectFeedthrough  VirtualResistor=DiscreDampingFlag  EquiInitial=true  ElecPortIOs=[ 1, 2 ]  SimulateUsing=Code generation
      mask Type: SimplusGT.Class.PhotovoltaicGFM
      mask Display:
      | disp('PhotovoltaicGFM');
      | port_label('input',1,'u');
      | port_label('output',1,'y');
  Math Function2 : Math  Operator=mod  SignedPower=on  SaturateOnIntegerOverflow=on
  Mux : Mux  Inputs=2
  Mux1 : Mux  Inputs=3
  Mux2 : Mux  Inputs=3
  Mux3 : Mux  Inputs=3
  PQ Calculation (dq-Frame) : Subsystem  AncestorBlock=|
      | SimplusGT/PQ Calculation
      | (dq-Frame)
  R_VD : spsThreePhaseSeriesRLCBranchLib/Three-Phase Series RLC Branch  LConnTagsString=A|B|C  RConnTagsString=A|B|C  BranchType=R  Resistance=DiscreDampingValue*Vbase^2/Sbase  Inductance=1e-3  Capacitance=1e-6  Measurements=None
  "abc -> dq (Power-Invariant)" : Subsystem  AncestorBlock=|
      | SimplusGT/abc -> dq
      | (Power-Invariant)
  "abc -> dq (Power-Invariant)1" : Subsystem  AncestorBlock=|
      | SimplusGT/abc -> dq
      | (Power-Invariant)
  "dq -> abc (Power-Invariant)" : Subsystem  AncestorBlock=|
      | SimplusGT/dq -> abc
      | (Power-Invariant)
  ia : spsControlledCurrentSourceLib/Controlled Current Source  Initialize=on  Source_Type=AC  Amplitude=0  Phase=0  Frequency=0  Measurements=None
  ia_m : spsCurrentMeasurementLib/Current Measurement  PhasorSimulation=off  OutputType=Complex  PSBequivalent=0
  ib : spsControlledCurrentSourceLib/Controlled Current Source  Initialize=on  Source_Type=AC  Amplitude=0  Phase=0  Frequency=0  Measurements=None
  ib_m : spsCurrentMeasurementLib/Current Measurement  PhasorSimulation=off  OutputType=Complex  PSBequivalent=0
  ic : spsControlledCurrentSourceLib/Controlled Current Source  Initialize=on  Source_Type=AC  Amplitude=0  Phase=0  Frequency=0  Measurements=None
  ic_m : spsCurrentMeasurementLib/Current Measurement  PhasorSimulation=off  OutputType=Complex  PSBequivalent=0
  va : spsVoltageMeasurementLib/Voltage Measurement  PhasorSimulation=off  OutputType=Complex  PSBequivalent=0
  vb : spsVoltageMeasurementLib/Voltage Measurement  PhasorSimulation=off  OutputType=Complex  PSBequivalent=0
  vc : spsVoltageMeasurementLib/Voltage Measurement  PhasorSimulation=off  OutputType=Complex  PSBequivalent=0
  a : PMIOPort  Side=Left
  b : PMIOPort  Port=2  Side=Left
  c : PMIOPort  Port=3  Side=Left
  n : PMIOPort  Port=4  Side=Left
  m : Outport
  wires:
  "abc -> dq (Power-Invariant)1"/1(dq) -> [i_dq_t]
  [theta] -> "abc -> dq (Power-Invariant)1"/2(theta)
  [i_abc_t] -> "abc -> dq (Power-Invariant)1"/1(abc)
  Mux3/1 -> Gain3/1
  Gain3/1 -> [i_abc_t]
  ib_m/1 -> Mux3/2
  ia_m/1 -> Mux3/1
  ic_m/1 -> Mux3/3
  Constant/1 -> Mux2/3
  Demux/4 -> Math Function2/1
  [v_dc] -> Bus Creator/8  "v_dc"
  Gain1/1 -> [v_abc]
  Gain2/1 -> Demux1/1
  PQ Calculation (dq-Frame)/1(pq) -> [pq]
  [i_dq_t] -> PQ Calculation (dq-Frame)/2(idq)  "i_dq"
  [v_dq] -> PQ Calculation (dq-Frame)/1(vdq)  "v_dq"
  [pq] -> Bus Creator/7  "pq"
  [i_abc] -> Gain2/1
  Gain/1 -> Bus Creator/5  "w"
  [w] -> Gain/1  "w"
  Bus Creator/1 -> m/1
  Math Function2/1 -> [theta]
  Constant5/1 -> Math Function2/2
  Demux1/3 -> ic/1
  vc/1 -> Mux1/3
  MATLAB System/1 -> Demux/1
  Mux2/1 -> MATLAB System/1
  "dq -> abc (Power-Invariant)"/1(abc) -> [i_abc]
  [theta] -> "dq -> abc (Power-Invariant)"/2(theta)
  [i_dq] -> "dq -> abc (Power-Invariant)"/1(dq)
  "abc -> dq (Power-Invariant)"/1(dq) -> [v_dq]
  [theta] -> "abc -> dq (Power-Invariant)"/2(theta)
  [v_abc] -> "abc -> dq (Power-Invariant)"/1(abc)
  [theta] -> Bus Creator/6  "theta"
  [i_abc_t] -> Bus Creator/4  "i_abc"
  [v_abc] -> Bus Creator/3  "v_abc"
  [i_dq_t] -> Bus Creator/2  "i_dq"
  [v_dq] -> Bus Creator/1  "v_dq"
  Demux2/2 -> Mux2/2
  Demux2/1 -> Mux2/1
  [v_dq] -> Demux2/1
  Mux1/1 -> Gain1/1
  vb/1 -> Mux1/2
  va/1 -> Mux1/1
  Demux1/2 -> ib/1
  Demux1/1 -> ia/1
  Demux/3 -> [w]
  Mux/1 -> [i_dq]
  Demux/1 -> Mux/1
  Demux/2 -> Mux/2
  connections:
  ic_m/LConn1 -- c/RConn1
  ib_m/LConn1 -- b/RConn1
  ia_m/LConn1 -- a/RConn1
  vc/LConn1 -- ic_m/RConn1 -- ic/LConn1 -- R_VD/LConn3
  ib/LConn1 -- vb/LConn1 -- ib_m/RConn1 -- R_VD/LConn2
  ia/LConn1 -- ia_m/RConn1 -- va/LConn1 -- R_VD/LConn1
  n/RConn1 -- ib/RConn1 -- ia/RConn1 -- ic/RConn1 -- R_VD/RConn1 -- R_VD/RConn2 -- R_VD/RConn3 -- vc/LConn2 -- va/LConn2 -- vb/LConn2

== system SimplusGT_2020a/ReIm2Complex ==
  note: Transformation from real/imaginary to complex vectors
      |
      | Author(s): Yitong Li
      |
      | Notes:
      |
      | A example is from dq frame to dq+- frame.
  Re Im : Inport
  -> backward : Fcn  Expr=u[1] - u[2]*1i
  -> forward : Fcn  Expr=u[1] + u[2]*1i
  Mux : Mux  Inputs=2
  +- : Outport
  wires:
  Re Im/1 -> -> backward/1, -> forward/1
  Mux/1 -> +-/1
  -> forward/1 -> Mux/1
  -> backward/1 -> Mux/2

== system SimplusGT_2020a/Root Mean Squre ==
  note: Root mean squre
      |
      | Author(s): Yitong Li
  x : Inport
  y : Inport  Port=2
  Math Function1 : Math  Operator=square  SignedPower=on  SaturateOnIntegerOverflow=on
  Math Function2 : Math  Operator=square  SignedPower=on  SaturateOnIntegerOverflow=on
  Sqrt : Sqrt  SaturateOnIntegerOverflow=on
  Sum : Sum
  RMS : Outport
  wires:
  Sum/1 -> Sqrt/1
  x/1 -> Math Function1/1
  Sqrt/1 -> RMS/1
  Math Function1/1 -> Sum/1
  y/1 -> Math Function2/1
  Math Function2/1 -> Sum/2

== system SimplusGT_2020a/Single Pulse ==
  note: Pulse generator
      |
      | Author(s): Yitong Li
  Gain : Gain  Gain=Am
  Product : Product
  Step : Step  Time=t0  SampleTime=0
  Step1 : Step  Time=t0+dt  Before=1  After=0  SampleTime=0
  Out : Outport
  wires:
  Step1/1 -> Product/2
  Step/1 -> Product/1
  Product/1 -> Gain/1
  Gain/1 -> Out/1
